simulink model "dc_motor"  (R2017b)
settings: Solver=VariableStepAuto  StartTime=0.0  StopTime=3  RelTol=1e-3
values from neighbouring files (symbols this model uses):
  B = Bm + Bl    (= 4.95148711841e-06)    [dc_motor_model.m]
  J = Jm + Jl    (= 1.3e-06)    [dc_motor_model.m]
  Ke = Rated_voltage / (No_load_speed)    (= 0.0238732414638)    [dc_motor_model.m]
  Kt = Rated_load / (Rated_load_current - No_load_current)    (= 0.0177777777778)    [dc_motor_model.m]
  L = 70e-6    (= 7e-05)    [dc_motor_model.m]
  Period = 2000    [dc_motor_model.m]
  R = 14.5    [dc_motor_model.m]
  r = 7e-3    (= 0.007)    [dc_motor_model.m]
  Text = 0    [dc_motor_model.m]
  V = 2.2    [dc_motor_model.m]
settings Model: Creator=Koen Schaper  LastModifiedBy=Koen Schaper

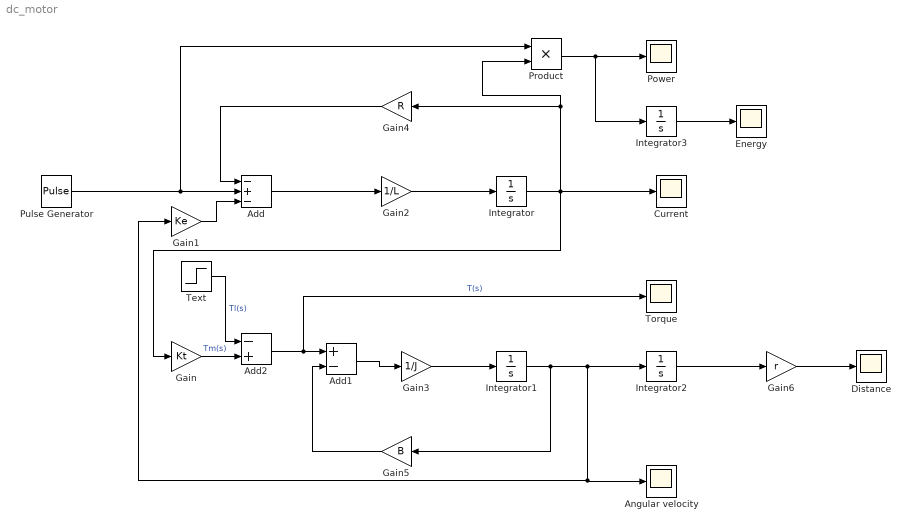
== system dc_motor ==
  Add : Sum  Inputs=-+-
  Add1 : Sum  Inputs=+-
  Add2 : Sum  Inputs=-+
  "Angular velocity " : Scope
  "Current " : Scope
      settings: Description=Current
  Distance : Scope
  Energy : Scope
  Gain : Gain  Gain=Kt
  Gain1 : Gain  Gain=Ke
  Gain2 : Gain  Gain=1/L
  Gain3 : Gain  Gain=1/J
  Gain4 : Gain  Gain=R
  Gain5 : Gain  Gain=B
  Gain6 : Gain  Gain=r
  Integrator{,1..3} (4 alike) : Integrator
  Power : Scope
  Product : Product
  Pulse Generator : DiscretePulseGenerator  PulseType=Time based  Amplitude=V  Period=1/Period  PulseWidth=30  PhaseDelay=1
  Text : Step  After=Text  SampleTime=0
  "Torque " : Scope
      settings: Description=Current
  wires:
  Add/1 -> Gain2/1
  Gain2/1 -> Integrator/1
  Pulse Generator/1 -> Product/1, Add/2
  Gain1/1 -> Add/3
  Gain/1 -> Add2/2  "Tm(s)"
  Gain4/1 -> Add/1
  Gain5/1 -> Add1/2
  Gain3/1 -> Integrator1/1
  Add1/1 -> Gain3/1
  Product/1 -> Integrator3/1, Power/1
  Add2/1 -> "Torque "/1, Add1/1  "T(s)"
  Text/1 -> Add2/1  "Tl(s)"
  Integrator1/1 -> Integrator2/1, Gain1/1, "Angular velocity "/1, Gain5/1
  Integrator/1 -> "Current "/1, Gain/1, Product/2, Gain4/1
  Integrator2/1 -> Gain6/1
  Gain6/1 -> Distance/1
  Integrator3/1 -> Energy/1
